simulink model "LIF_Neuron_Model"  (R2023b)
settings: Solver=FixedStepAuto  StartTime=0.0  StopTime=0.5  FixedStep=h  RelTol=1e-3
values from neighbouring files (symbols this model uses):
  E_e = 0    [Improved_Network_Constants.m]    (also in LIF_Neuron_Constants.m)
  E_i = -70    [Improved_Network_Constants.m]    (also in LIF_Neuron_Constants.m)
  g_lut = g(lut_indices)*1000    [Improved_Network_Constants.m]    (also in LIF_Neuron_Constants.m)
  h = 0.0001    [Improved_Network_Constants.m]    (also in LIF_Neuron_Constants.m)
  Rm = 20*10^-2    (= 0.2)    [Improved_Network_Constants.m]    (also in LIF_Neuron_Constants.m)
  tao_m = 50*10^-3    (= 0.05)    [Improved_Network_Constants.m]    (also in LIF_Neuron_Constants.m)
  V_thr = -50    [Improved_Network_Constants.m]    (also in LIF_Neuron_Constants.m)
  Vo = -65    [Improved_Network_Constants.m]    (also in LIF_Neuron_Constants.m)
libraries: hdlsllib x4
settings Model: Creator=Sertan  LastModifiedBy=Sertan
settings OptimizationCC: BlockReduction=off  ConditionallyExecuteInputs=off

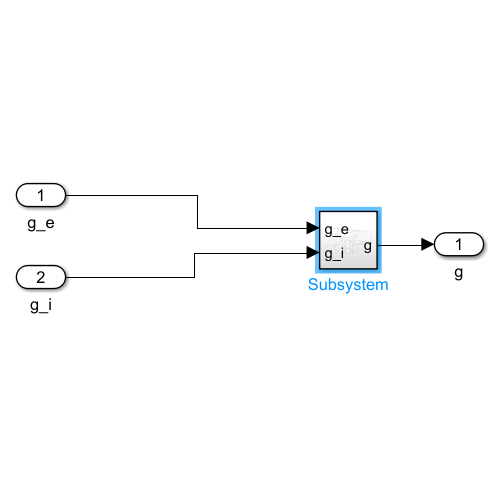
[thumbnail: Simulink's stored preview of the top-level diagram]
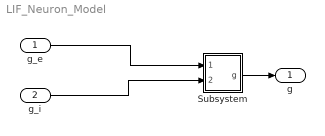
== system LIF_Neuron_Model ==
  g_e : Inport
  g_i : Inport  Port=2
  Subsystem : Subsystem
  g : Outport  VectorParamsAs1DForOutWhenUnconnected=off
  wires:
  g_i/1 -> Subsystem/2(g_i)
  g_e/1 -> Subsystem/1(g_e)
  Subsystem/1(g) -> g/1

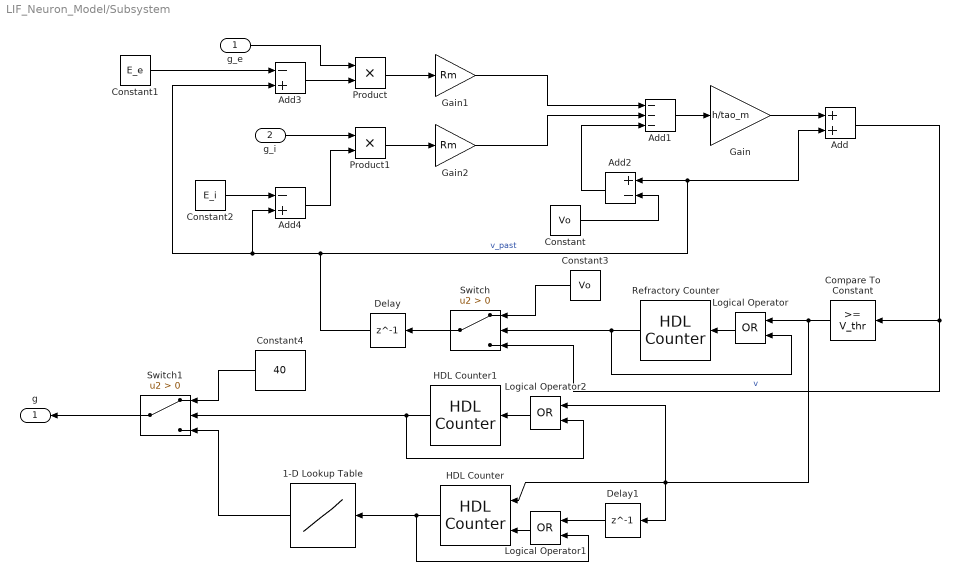
== system LIF_Neuron_Model/Subsystem ==
  g_e : Inport
  g_i : Inport  Port=2
  1-D Lookup Table : Lookup_n-D  NumberOfTableDimensions=1  LookupTableObject=''  BreakpointsForDimension1=[0:201]  BreakpointsForDimension1FirstPoint=10  BreakpointsForDimension2FirstPoint=10  BreakpointsForDimension1Spacing=12  BreakpointsForDimension2Spacing=12  BreakpointsForDimension1DataTypeStr=Inherit: Inherit from 'Breakpoint data'  IndexSearchMethod=Evenly spaced points  Table=g_lut  InterpMethod=Flat  DiagnosticForOutOfRangeInput=Error  InternalRulePriority=Speed  OutDataTypeStr=fixdt(1,16,8)  RndMeth=Simplest
  Add : Sum
  Add1 : Sum  Inputs=---
  Add2 : Sum  Inputs=+-
  Add3 : Sum  Inputs=-+
  Add4 : Sum  Inputs=-+
  Compare To Constant : hdlsllib/Logic and Bit Operations/Compare To Constant  relop=>=  const=V_thr  OutDataTypeStr=boolean
  Constant : Constant  Value=Vo  OutDataTypeStr=fixdt(1,16,8)
  Constant1 : Constant  Value=E_e  OutDataTypeStr=fixdt(1,16,8)
  Constant2 : Constant  Value=E_i  OutDataTypeStr=fixdt(1,16,8)
  Constant3 : Constant  Value=Vo  OutDataTypeStr=fixdt(1,16,8)
  Constant4 : Constant  Value=40  OutDataTypeStr=fixdt(1,16,8)
  Delay : Delay  DelayLength=1  InitialCondition=Vo
  Delay1 : Delay  DelayLength=1  InitialCondition=0
  Gain : Gain  Gain=h/tao_m  OutDataTypeStr=fixdt(1,16,8)
  Gain1 : Gain  Gain=Rm
  Gain2 : Gain  Gain=Rm
  HDL Counter : hdlsllib/Sources/HDL Counter  CountType=Count limited  CountInit=0  CountStep=1  CountMax=length(g_lut)-1  CountFromType=Initial value  CountFrom=0  CountResetPort=on  CountLoadPort=off  CountEnbPort=on  CountDirPort=off  CountHitOutputPort=off  CountDataType=Unsigned  CountWordLen=8  CountFracLen=0  CountSampTime=1
  HDL Counter1 : hdlsllib/Sources/HDL Counter  CountType=Count limited  CountInit=0  CountStep=1  CountMax=2  CountFromType=Initial value  CountFrom=0  CountResetPort=off  CountLoadPort=off  CountEnbPort=on  CountDirPort=off  CountHitOutputPort=off  CountDataType=Unsigned  CountWordLen=8  CountFracLen=0  CountSampTime=1
  Logical Operator : Logic  Operator=OR  AllPortsSameDT=off  OutDataTypeStr=boolean
  Logical Operator1 : Logic  Operator=OR  AllPortsSameDT=off  OutDataTypeStr=boolean
  Logical Operator2 : Logic  Operator=OR  AllPortsSameDT=off  OutDataTypeStr=boolean
  Product : Product
  Product1 : Product
  Refractory Counter : hdlsllib/Sources/HDL Counter  CountType=Count limited  CountInit=0  CountStep=1  CountMax=r_time  CountFromType=Initial value  CountFrom=0  CountResetPort=off  CountLoadPort=off  CountEnbPort=on  CountDirPort=off  CountHitOutputPort=off  CountDataType=Unsigned  CountWordLen=8  CountFracLen=0  CountSampTime=1
  Switch : Switch  Criteria=u2 > Threshold  SaturateOnIntegerOverflow=off  InputSameDT=off
  Switch1 : Switch  Criteria=u2 > Threshold  OutDataTypeStr=fixdt(1,16,8)  SaturateOnIntegerOverflow=off  InputSameDT=off
  g : Outport  VectorParamsAs1DForOutWhenUnconnected=off
  wires:
  Constant/1 -> Add2/2
  Delay/1 -> Add3/2, Add4/2, Add/2, Add2/1  "v_past"
  Add/1 -> Switch/3, Compare To Constant/1  "v"
  g_i/1 -> Product1/1
  Gain1/1 -> Add1/1
  Add2/1 -> Add1/3
  Add1/1 -> Gain/1
  Add4/1 -> Product1/2
  Product/1 -> Gain1/1
  Add3/1 -> Product/2
  Gain2/1 -> Add1/2
  Gain/1 -> Add/1
  g_e/1 -> Product/1
  Constant1/1 -> Add3/1
  Constant2/1 -> Add4/1
  Product1/1 -> Gain2/1
  Constant3/1 -> Switch/1
  Refractory Counter/1 -> Logical Operator/2, Switch/2
  Logical Operator/1 -> Refractory Counter/1
  HDL Counter/1 -> Logical Operator1/2, 1-D Lookup Table/1
  Switch1/1 -> g/1
  Switch/1 -> Delay/1
  1-D Lookup Table/1 -> Switch1/3
  Logical Operator1/1 -> HDL Counter/2
  Delay1/1 -> Logical Operator1/1
  Constant4/1 -> Switch1/1
  Logical Operator2/1 -> HDL Counter1/1
  HDL Counter1/1 -> Switch1/2, Logical Operator2/2
  Compare To Constant/1 -> Logical Operator/1, Delay1/1, Logical Operator2/1, HDL Counter/1
